simulink model "Cell_model_final3"  (R2023a)
settings: Solver=VariableStepAuto  StartTime=0.0  StopTime=T_e  RelTol=1e-3
values from neighbouring files (symbols this model uses):
  C1_253 = zeros(1,11)+1000    [for_the_new_parameter_estimator.m]
  C1_263 = zeros(1,11)+1000    [for_the_new_parameter_estimator.m]
  C1_273 = zeros(1,11)+1000    [for_the_new_parameter_estimator.m]
  C1_283 = zeros(1,11)+1000    [for_the_new_parameter_estimator.m]
  C1_298 = zeros(1,11)+1000    [for_the_new_parameter_estimator.m]
  OCV_253 = zeros(1,11)+4    [for_the_new_parameter_estimator.m]
  OCV_263 = zeros(1,11)+4    [for_the_new_parameter_estimator.m]
  OCV_273 = zeros(1,11)+4    [for_the_new_parameter_estimator.m]
  OCV_283 = zeros(1,11)+4    [for_the_new_parameter_estimator.m]
  OCV_298 = zeros(1,11)+4    [for_the_new_parameter_estimator.m]
  R0_253 = zeros(1,11)    [for_the_new_parameter_estimator.m]
  R0_263 = zeros(1,11)    [for_the_new_parameter_estimator.m]
  R0_273 = zeros(1,11)    [for_the_new_parameter_estimator.m]
  R0_283 = zeros(1,11)    [for_the_new_parameter_estimator.m]
  R0_298 = zeros(1,11)    [for_the_new_parameter_estimator.m]
  R1_253 = zeros(1,11)    [for_the_new_parameter_estimator.m]
  R1_263 = zeros(1,11)    [for_the_new_parameter_estimator.m]
  R1_273 = zeros(1,11)    [for_the_new_parameter_estimator.m]
  R1_283 = zeros(1,11)    [for_the_new_parameter_estimator.m]
  R1_298 = zeros(1,11)    [for_the_new_parameter_estimator.m]
libraries: neural x100, fl_lib x11, nesl_utility x11, BatteryEstimators x1, ee_lib x1, spspowerguiLib x1
(part 4 of 4)

== system Cell_model_final3/Battery/Subsystem/Custom Neural Network1/Layer 5/Delays 1 ==
  "p{5}" : Inport  PortDimensions=10
      mask Display: e = 0.06;c1 = [120 230 180]/255;c2 = ([120 230 180]+0)/(256+128);c3 = ([120 230 180]+128)/(256+128);patch([0 1 1 0],[0 0 1 1],c1);patch([0 1 1 1-e 1-e 0+e],[0 0 1 1-e 0+e 0+e],c2);patch([0 0 1 1-e 0+e 0+e],[0 1 1 1-e 1-e 0+e],c3);plot([0 1 1 0 0],[0 0 1 1 0]);
  mux : Mux  Inputs=1
      mask Display: e = 0.06;c1 = [120 150 230]/255;c2 = ([120 150 230]+0)/383;c3 = ([120 150 230]+128)/383;patch([0 1 1 0],[0 0 1 1],c1);patch([0 1 1 1-e 1-e 0+e],[0 0 1 1-e 0+e 0+e],c2);patch([0 0 1 1-e 0+e 0+e],[0 1 1 1-e 1-e 0+e],c3);plot([0 1 1 0 0],[0 0 1 1 0]);disp('Mux')
  "pd{5,4}" : Outport
      mask Display: e = 0.06;c1 = [120 230 180]/255;c2 = ([120 230 180]+0)/(256+128);c3 = ([120 230 180]+128)/(256+128);patch([0 1 1 0],[0 0 1 1],c1);patch([0 1 1 1-e 1-e 0+e],[0 0 1 1-e 0+e 0+e],c2);patch([0 0 1 1-e 0+e 0+e],[0 1 1 1-e 1-e 0+e],c3);plot([0 1 1 0 0],[0 0 1 1 0]);
  wires:
  "p{5}"/1 -> mux/1
  mux/1 -> "pd{5,4}"/1

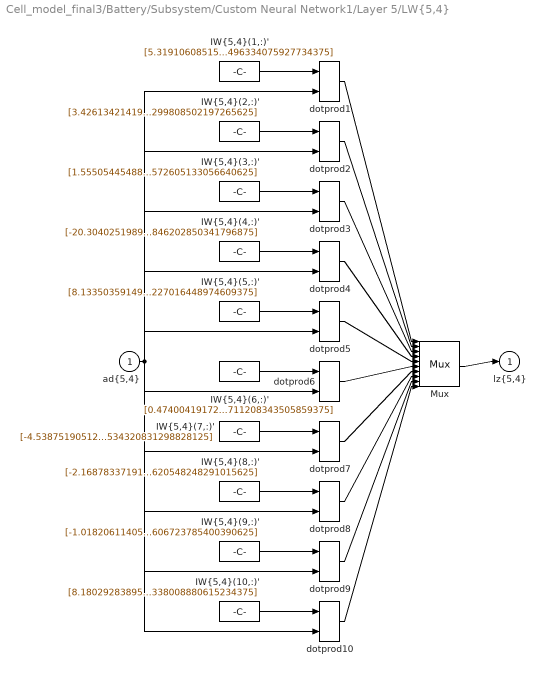
== system Cell_model_final3/Battery/Subsystem/Custom Neural Network1/Layer 5/LW{5,4} ==
  "ad{5,4}" : Inport  PortDimensions=10
      mask Display: e = 0.06;c1 = [120 230 180]/255;c2 = ([120 230 180]+0)/(256+128);c3 = ([120 230 180]+128)/(256+128);patch([0 1 1 0],[0 0 1 1],c1);patch([0 1 1 1-e 1-e 0+e],[0 0 1 1-e 0+e 0+e],c2);patch([0 0 1 1-e 0+e 0+e],[0 1 1 1-e 1-e 0+e],c3);plot([0 1 1 0 0],[0 0 1 1 0]);
  "IW{5,4}(1,:)'" : Constant  Value=[5.31910608515874283597213434404693543910980224609375;-37.6187219247760680218561901710927486419677734375;-1.434327602098746989867095180670730769634246826171875;-1.3067931540625294939417244677315466105937957763671875;0.08338336636821926106666325040350784547626972198486328125;3.10444042714829127049824819550849497318267822265625;3.20260944459612328927278213086538016796112060546875;0.69515320195009311365907933577545918524265289306640625;1.22868083139611439236205114866606891155242919921875;-5.956084539158521096169351949356496334075927734375]
      mask Display: e = 0.06;c1 = [120 150 230]/255;c2 = ([120 150 230]+0)/383;c3 = ([120 150 230]+128)/383;patch([0 1 1 0],[0 0 1 1],c1);patch([0 1 1 1-e 1-e 0+e],[0 0 1 1-e 0+e 0+e],c2);patch([0 0 1 1-e 0+e 0+e],[0 1 1 1-e 1-e 0+e],c3);plot([0 1 1 0 0],[0 0 1 1 0]);disp('weights');
  "IW{5,4}(10,:)'" : Constant  Value=[8.18029283895581471597324707545340061187744140625;-0.86604032375827444401039656440843828022480010986328125;10.406226965972205533716987702064216136932373046875;-8.485710592220481629510686616413295269012451171875;-0.251726104378499015989945064575294964015483856201171875;20.0634977846928421740813064388930797576904296875;-1.366718568608316086709919545683078467845916748046875;27.82724288856896777133442810736596584320068359375;4.8484804648080181976865787873975932598114013671875;3.57714877656545038320246021612547338008880615234375]
      mask Display: e = 0.06;c1 = [120 150 230]/255;c2 = ([120 150 230]+0)/383;c3 = ([120 150 230]+128)/383;patch([0 1 1 0],[0 0 1 1],c1);patch([0 1 1 1-e 1-e 0+e],[0 0 1 1-e 0+e 0+e],c2);patch([0 0 1 1-e 0+e 0+e],[0 1 1 1-e 1-e 0+e],c3);plot([0 1 1 0 0],[0 0 1 1 0]);disp('weights');
  "IW{5,4}(2,:)'" : Constant  Value=[3.42613421419545005619511357508599758148193359375;1.114618823772122624404801172204315662384033203125;-6.75680619223893419444948449381627142429351806640625;-1.91855581646149797592215691111050546169281005859375;-3.572382975305118169018214757670648396015167236328125;4.45780515936019838818538119085133075714111328125;-5.79158021666007538641451901639811694622039794921875;4.38311052670753742432907529291696846485137939453125;-1.7471431694872290307785078766755759716033935546875;-1.199354747415134259114211090491153299808502197265625]
      mask Display: e = 0.06;c1 = [120 150 230]/255;c2 = ([120 150 230]+0)/383;c3 = ([120 150 230]+128)/383;patch([0 1 1 0],[0 0 1 1],c1);patch([0 1 1 1-e 1-e 0+e],[0 0 1 1-e 0+e 0+e],c2);patch([0 0 1 1-e 0+e 0+e],[0 1 1 1-e 1-e 0+e],c3);plot([0 1 1 0 0],[0 0 1 1 0]);disp('weights');
  "IW{5,4}(3,:)'" : Constant  Value=[1.555054454884164716332861644332297146320343017578125;0.280436030021297078018704951318795792758464813232421875;-1.340061650945262083922671081381849944591522216796875;1.6251508867869788321769419781048782169818878173828125;-1.0157386511680421836700816129450686275959014892578125;-5.35130459212175946248635227675549685955047607421875;0.76519595505605464413889649222255684435367584228515625;0.2585494067780447213777961223968304693698883056640625;0.7317476832289095955985658292775042355060577392578125;-1.637176688866903706554012387641705572605133056640625]
      mask Display: e = 0.06;c1 = [120 150 230]/255;c2 = ([120 150 230]+0)/383;c3 = ([120 150 230]+128)/383;patch([0 1 1 0],[0 0 1 1],c1);patch([0 1 1 1-e 1-e 0+e],[0 0 1 1-e 0+e 0+e],c2);patch([0 0 1 1-e 0+e 0+e],[0 1 1 1-e 1-e 0+e],c3);plot([0 1 1 0 0],[0 0 1 1 0]);disp('weights');
  "IW{5,4}(4,:)'" : Constant  Value=[-20.30402519890122903234441764652729034423828125;22.457629621246137929801989230327308177947998046875;0.314878492933852116575366153483628295361995697021484375;-44.36293643056806246249834657646715641021728515625;7.3827011574238969870975779485888779163360595703125;-35.88281999329792171238295850344002246856689453125;60.188644212525076682140934281051158905029296875;-8.9725237313902770353024607175029814243316650390625;-7.32605500412379928576456222799606621265411376953125;20.154382584722309701419362681917846202850341796875]
      mask Display: e = 0.06;c1 = [120 150 230]/255;c2 = ([120 150 230]+0)/383;c3 = ([120 150 230]+128)/383;patch([0 1 1 0],[0 0 1 1],c1);patch([0 1 1 1-e 1-e 0+e],[0 0 1 1-e 0+e 0+e],c2);patch([0 0 1 1-e 0+e 0+e],[0 1 1 1-e 1-e 0+e],c3);plot([0 1 1 0 0],[0 0 1 1 0]);disp('weights');
  "IW{5,4}(5,:)'" : Constant  Value=[8.1335035914949518343064482905901968479156494140625;15.49384820678261576176737435162067413330078125;37.736545982073863569894456304609775543212890625;-13.3628093022243650267455450375564396381378173828125;-8.62393036572091631342118489556014537811279296875;-16.40819498321757663461539777927100658416748046875;-3.410303327601974299199127926840446889400482177734375;24.133962885927786601314437575638294219970703125;-16.080026613818450442749963258393108844757080078125;9.37803262099551915298434323631227016448974609375]
      mask Display: e = 0.06;c1 = [120 150 230]/255;c2 = ([120 150 230]+0)/383;c3 = ([120 150 230]+128)/383;patch([0 1 1 0],[0 0 1 1],c1);patch([0 1 1 1-e 1-e 0+e],[0 0 1 1-e 0+e 0+e],c2);patch([0 0 1 1-e 0+e 0+e],[0 1 1 1-e 1-e 0+e],c3);plot([0 1 1 0 0],[0 0 1 1 0]);disp('weights');
  "IW{5,4}(6,:)'" : Constant  Value=[0.474004191724247625483457113659824244678020477294921875;-0.771879334027128383155513802194036543369293212890625;1.25980116172532152774010683060623705387115478515625;5.09481225898411604902094040880911052227020263671875;-6.057666156447250926930792047642171382904052734375;1.0032813129573601163002649627742357552051544189453125;0.54980960210650720032532490222365595400333404541015625;5.677288355257385177310425206087529659271240234375;3.371131008149129026918444651528261601924896240234375;0.339900525159732236346599165699444711208343505859375]
      mask Display: e = 0.06;c1 = [120 150 230]/255;c2 = ([120 150 230]+0)/383;c3 = ([120 150 230]+128)/383;patch([0 1 1 0],[0 0 1 1],c1);patch([0 1 1 1-e 1-e 0+e],[0 0 1 1-e 0+e 0+e],c2);patch([0 0 1 1-e 0+e 0+e],[0 1 1 1-e 1-e 0+e],c3);plot([0 1 1 0 0],[0 0 1 1 0]);disp('weights');
  "IW{5,4}(7,:)'" : Constant  Value=[-4.53875190512472048709469163441099226474761962890625;-1.27624362940507030117487374809570610523223876953125;-0.5325326436101438520864803649601526558399200439453125;-0.76454466657364406056984762471984140574932098388671875;1.3293898148616258847454218994244001805782318115234375;8.2016192404383243541587944491766393184661865234375;-0.420980338568227863138559996514231897890567779541015625;-0.32581960761651063140931228190311230719089508056640625;3.68923545619525139471761576714925467967987060546875;3.654730298709310876148492752690799534320831298828125]
      mask Display: e = 0.06;c1 = [120 150 230]/255;c2 = ([120 150 230]+0)/383;c3 = ([120 150 230]+128)/383;patch([0 1 1 0],[0 0 1 1],c1);patch([0 1 1 1-e 1-e 0+e],[0 0 1 1-e 0+e 0+e],c2);patch([0 0 1 1-e 0+e 0+e],[0 1 1 1-e 1-e 0+e],c3);plot([0 1 1 0 0],[0 0 1 1 0]);disp('weights');
  "IW{5,4}(8,:)'" : Constant  Value=[-2.1687833719175610980300916708074510097503662109375;-1.555262101477545844119276807759888470172882080078125;3.63732074692894880030280546634458005428314208984375;-2.926721780427193220219805880333296954631805419921875;-3.199812050957930420480579414288513362407684326171875;3.306279673153628362314293553936295211315155029296875;-1.710894450984811410165775669156573712825775146484375;-0.958158604621420550984112196601927280426025390625;1.156343479755686853849283579620532691478729248046875;6.4019059577235708502485067583620548248291015625]
      mask Display: e = 0.06;c1 = [120 150 230]/255;c2 = ([120 150 230]+0)/383;c3 = ([120 150 230]+128)/383;patch([0 1 1 0],[0 0 1 1],c1);patch([0 1 1 1-e 1-e 0+e],[0 0 1 1-e 0+e 0+e],c2);patch([0 0 1 1-e 0+e 0+e],[0 1 1 1-e 1-e 0+e],c3);plot([0 1 1 0 0],[0 0 1 1 0]);disp('weights');
  "IW{5,4}(9,:)'" : Constant  Value=[-1.018206114054226230081212634104304015636444091796875;0.049203477607104494084833135048029362224042415618896484375;1.100856722356188921452258000499568879604339599609375;-0.048629482677228268172608949271307210437953472137451171875;-0.353114170971075946869888184664887376129627227783203125;-0.09062537123318527287896273492151522077620029449462890625;-0.77821592155081731334576033987104892730712890625;-0.208814446511384643745401490377844311296939849853515625;-0.6086582230673425186751046567223966121673583984375;1.30310740687895876277480056160129606723785400390625]
      mask Display: e = 0.06;c1 = [120 150 230]/255;c2 = ([120 150 230]+0)/383;c3 = ([120 150 230]+128)/383;patch([0 1 1 0],[0 0 1 1],c1);patch([0 1 1 1-e 1-e 0+e],[0 0 1 1-e 0+e 0+e],c2);patch([0 0 1 1-e 0+e 0+e],[0 1 1 1-e 1-e 0+e],c3);plot([0 1 1 0 0],[0 0 1 1 0]);disp('weights');
  Mux : Mux  Inputs=10
      mask Display: e = 0.06;c1 = [120 150 230]/255;c2 = ([120 150 230]+0)/383;c3 = ([120 150 230]+128)/383;patch([0 1 1 0],[0 0 1 1],c1);patch([0 1 1 1-e 1-e 0+e],[0 0 1 1-e 0+e 0+e],c2);patch([0 0 1 1-e 0+e 0+e],[0 1 1 1-e 1-e 0+e],c3);plot([0 1 1 0 0],[0 0 1 1 0]);disp('Mux');
  dotprod{1..10} (10 alike) : neural/Weight Functions/dotprod
  "lz{5,4}" : Outport
      mask Display: e = 0.06;c1 = [120 230 180]/255;c2 = ([120 230 180]+0)/(256+128);c3 = ([120 230 180]+128)/(256+128);patch([0 1 1 0],[0 0 1 1],c1);patch([0 1 1 1-e 1-e 0+e],[0 0 1 1-e 0+e 0+e],c2);patch([0 0 1 1-e 0+e 0+e],[0 1 1 1-e 1-e 0+e],c3);plot([0 1 1 0 0],[0 0 1 1 0]);
  wires:
  "IW{5,4}(1,:)'"/1 -> dotprod1/1
  "ad{5,4}"/1 -> dotprod1/2, dotprod2/2, dotprod3/2, dotprod4/2, dotprod5/2, dotprod6/2, dotprod7/2, dotprod8/2, dotprod9/2, dotprod10/2
  dotprod1/1 -> Mux/1
  "IW{5,4}(2,:)'"/1 -> dotprod2/1
  dotprod2/1 -> Mux/2
  "IW{5,4}(3,:)'"/1 -> dotprod3/1
  dotprod3/1 -> Mux/3
  "IW{5,4}(4,:)'"/1 -> dotprod4/1
  dotprod4/1 -> Mux/4
  "IW{5,4}(5,:)'"/1 -> dotprod5/1
  dotprod5/1 -> Mux/5
  "IW{5,4}(6,:)'"/1 -> dotprod6/1
  dotprod6/1 -> Mux/6
  "IW{5,4}(7,:)'"/1 -> dotprod7/1
  dotprod7/1 -> Mux/7
  "IW{5,4}(8,:)'"/1 -> dotprod8/1
  dotprod8/1 -> Mux/8
  "IW{5,4}(9,:)'"/1 -> dotprod9/1
  dotprod9/1 -> Mux/9
  "IW{5,4}(10,:)'"/1 -> dotprod10/1
  dotprod10/1 -> Mux/10
  Mux/1 -> "lz{5,4}"/1

== system Cell_model_final3/Battery/Subsystem/Custom Neural Network1/Layer 6/Delays 1 ==
  "p{6}" : Inport  PortDimensions=10
      mask Display: e = 0.06;c1 = [120 230 180]/255;c2 = ([120 230 180]+0)/(256+128);c3 = ([120 230 180]+128)/(256+128);patch([0 1 1 0],[0 0 1 1],c1);patch([0 1 1 1-e 1-e 0+e],[0 0 1 1-e 0+e 0+e],c2);patch([0 0 1 1-e 0+e 0+e],[0 1 1 1-e 1-e 0+e],c3);plot([0 1 1 0 0],[0 0 1 1 0]);
  mux : Mux  Inputs=1
      mask Display: e = 0.06;c1 = [120 150 230]/255;c2 = ([120 150 230]+0)/383;c3 = ([120 150 230]+128)/383;patch([0 1 1 0],[0 0 1 1],c1);patch([0 1 1 1-e 1-e 0+e],[0 0 1 1-e 0+e 0+e],c2);patch([0 0 1 1-e 0+e 0+e],[0 1 1 1-e 1-e 0+e],c3);plot([0 1 1 0 0],[0 0 1 1 0]);disp('Mux')
  "pd{6,5}" : Outport
      mask Display: e = 0.06;c1 = [120 230 180]/255;c2 = ([120 230 180]+0)/(256+128);c3 = ([120 230 180]+128)/(256+128);patch([0 1 1 0],[0 0 1 1],c1);patch([0 1 1 1-e 1-e 0+e],[0 0 1 1-e 0+e 0+e],c2);patch([0 0 1 1-e 0+e 0+e],[0 1 1 1-e 1-e 0+e],c3);plot([0 1 1 0 0],[0 0 1 1 0]);
  wires:
  "p{6}"/1 -> mux/1
  mux/1 -> "pd{6,5}"/1

== system Cell_model_final3/Battery/Subsystem/Custom Neural Network1/Layer 6/LW{6,5} ==
  "ad{6,5}" : Inport  PortDimensions=10
      mask Display: e = 0.06;c1 = [120 230 180]/255;c2 = ([120 230 180]+0)/(256+128);c3 = ([120 230 180]+128)/(256+128);patch([0 1 1 0],[0 0 1 1],c1);patch([0 1 1 1-e 1-e 0+e],[0 0 1 1-e 0+e 0+e],c2);patch([0 0 1 1-e 0+e 0+e],[0 1 1 1-e 1-e 0+e],c3);plot([0 1 1 0 0],[0 0 1 1 0]);
  "IW{6,5}(1,:)'" : Constant  Value=[-0.406429640109170875472699435704271309077739715576171875;-0.267371167482458316211335613843402825295925140380859375;-0.71984747692384021267031357638188637793064117431640625;0.043158778961537129503778231764954398386180400848388671875;0.04783387904272039248265713240471086464822292327880859375;0.2008960714624491716850940292715677060186862945556640625;-0.40349557711881012256327494469587691128253936767578125;-0.2021370367535566814343184205426950938999652862548828125;-1.0259539320283483920803746514138765633106231689453125;-0.09320849323068969294325825103442184627056121826171875]
      mask Display: e = 0.06;c1 = [120 150 230]/255;c2 = ([120 150 230]+0)/383;c3 = ([120 150 230]+128)/383;patch([0 1 1 0],[0 0 1 1],c1);patch([0 1 1 1-e 1-e 0+e],[0 0 1 1-e 0+e 0+e],c2);patch([0 0 1 1-e 0+e 0+e],[0 1 1 1-e 1-e 0+e],c3);plot([0 1 1 0 0],[0 0 1 1 0]);disp('weights');
  Mux : Mux  Inputs=1
      mask Display: e = 0.06;c1 = [120 150 230]/255;c2 = ([120 150 230]+0)/383;c3 = ([120 150 230]+128)/383;patch([0 1 1 0],[0 0 1 1],c1);patch([0 1 1 1-e 1-e 0+e],[0 0 1 1-e 0+e 0+e],c2);patch([0 0 1 1-e 0+e 0+e],[0 1 1 1-e 1-e 0+e],c3);plot([0 1 1 0 0],[0 0 1 1 0]);disp('Mux');
  dotprod1 : neural/Weight Functions/dotprod
  "lz{6,5}" : Outport
      mask Display: e = 0.06;c1 = [120 230 180]/255;c2 = ([120 230 180]+0)/(256+128);c3 = ([120 230 180]+128)/(256+128);patch([0 1 1 0],[0 0 1 1],c1);patch([0 1 1 1-e 1-e 0+e],[0 0 1 1-e 0+e 0+e],c2);patch([0 0 1 1-e 0+e 0+e],[0 1 1 1-e 1-e 0+e],c3);plot([0 1 1 0 0],[0 0 1 1 0]);
  wires:
  "IW{6,5}(1,:)'"/1 -> dotprod1/1
  "ad{6,5}"/1 -> dotprod1/2
  dotprod1/1 -> Mux/1
  Mux/1 -> "lz{6,5}"/1

== matlab function Cell_model_final3/Battery/Subsystem/MATLAB Function ==
  data: u input; y output; v input; w input
function y = fcn(u,v,w)


all=[u;v;w];

y = all;
